simulink model "example_1_attitude_rate"  (R2016a)
settings: Solver=VariableStepAuto  StartTime=0.0  StopTime=Tsim  RelTol=1e-3
values from neighbouring files (symbols this model uses):
  ref_A = [10, 10, 10]    [init_A.m]    (also in init_B.m = [3, 6, 9])
  ref_b = [0, 0, 0]    [init_A.m]    (also in init_B.m)
  ref_p = [1, 2, 3]    [init_A.m]    (also in init_B.m = [pi/2, pi/2, pi/2])
  ref_w = [1, 2, 3]    [init_A.m]    (also in init_B.m = [0, 0, 0])
settings Model: Creator=mgreiff  LastModifiedBy=mgreiff

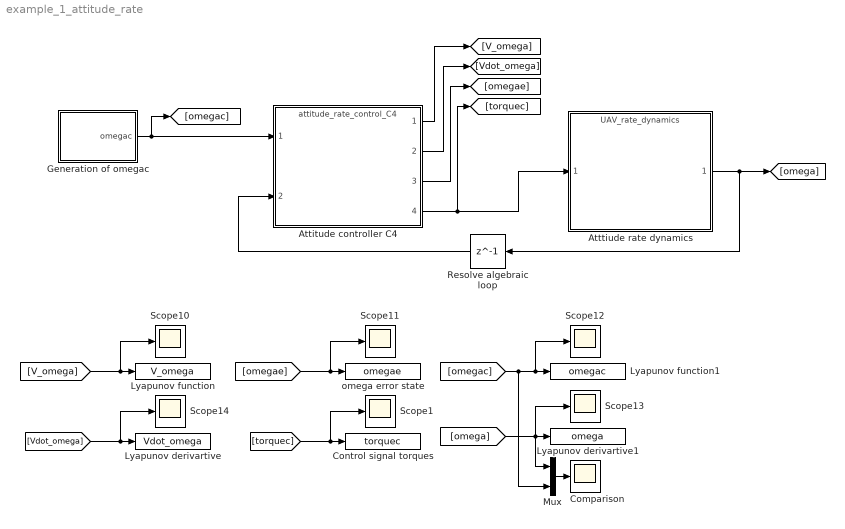
== system example_1_attitude_rate ==
  Attitude controller C4 : ModelReference  ModelNameDialog=attitude_rate_control_C4.slx  SimulationMode=Normal  ModelReferenceVersion=1.37
  Atttiude rate dynamics : ModelReference  ModelNameDialog=UAV_rate_dynamics.slx  SimulationMode=Normal  ModelReferenceVersion=1.9
  Comparison : Scope
  Control signal torques : ToWorkspace  VariableName=torquec  SaveFormat=Timeseries  SampleTime=-1
  Generation of omegac : Subsystem
  Lyapunov derivartive : ToWorkspace  VariableName=Vdot_omega  SaveFormat=Timeseries  SampleTime=-1
  Lyapunov derivartive1 : ToWorkspace  VariableName=omega  SaveFormat=Timeseries  SampleTime=-1
  Lyapunov function : ToWorkspace  VariableName=V_omega  SaveFormat=Timeseries  SampleTime=-1
  Lyapunov function1 : ToWorkspace  VariableName=omegac  SaveFormat=Timeseries  SampleTime=-1
  Mux : Mux  Inputs=2
  Resolve algebraic loop : Delay  DelayLength=1  InitialCondition=0  SampleTime=0.001
  Scope{1,10..14} (6 alike) : Scope
  omega error state : ToWorkspace  VariableName=omegae  SaveFormat=Timeseries  SampleTime=-1
  wires:
  Generation of omegac/1("omegac ") -> [omegac], Attitude controller C4/1
  [V_omega] -> Lyapunov function/1, Scope10/1
  [Vdot_omega] -> Lyapunov derivartive/1, Scope14/1
  [omegac] -> Mux/2, Lyapunov function1/1, Scope12/1
  [omega] -> Mux/1, Lyapunov derivartive1/1, Scope13/1
  [omegae] -> omega error state/1, Scope11/1
  Attitude controller C4/4 -> Atttiude rate dynamics/1, [torquec]
  Attitude controller C4/1 -> [V_omega]
  Attitude controller C4/2 -> [Vdot_omega]
  Attitude controller C4/3 -> [omegae]
  Mux/1 -> Comparison/1
  [torquec] -> Control signal torques/1, Scope1/1
  Atttiude rate dynamics/1 -> Resolve algebraic loop/1, [omega]
  Resolve algebraic loop/1 -> Attitude controller C4/2

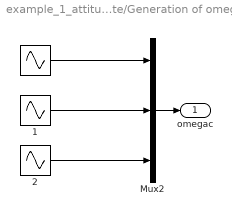
== system example_1_attitude_rate/Generation of omegac ==
  " " : Sin  Amplitude=ref_A(1)  Bias=ref_b(1)  Frequency=ref_w(1)  Phase=ref_p(1)  SampleTime=0.001
  " 1" : Sin  Amplitude=ref_A(2)  Bias=ref_b(2)  Frequency=ref_w(2)  Phase=ref_p(2)  SampleTime=0.001
  " 2" : Sin  Amplitude=ref_A(3)  Bias=ref_b(3)  Frequency=ref_w(3)  Phase=ref_p(3)  SampleTime=0.001
  Mux2 : Mux  Inputs=3
  "omegac " : Outport
  wires:
  Mux2/1 -> "omegac "/1
  " "/1 -> Mux2/1
  " 2"/1 -> Mux2/3
  " 1"/1 -> Mux2/2
